simulink model "SimpleBotModel"  (R2024a)
settings: Solver=ode15s  StartTime=0.0  StopTime=2  MaxStep=1e-3  MinStep=1e-5  RelTol=1e-6  AbsTol=1e-3
values from neighbouring files (symbols this model uses):
  Achsabstand = 0.15    [Model1Sensibilities.m]    (also in Model1numericalPSA.m; Model2Sensibilities.m; Modellvalidierung.m; MotorSens2.m)
  B_dis = 0.25    [Model1Sensibilities.m]    (also in Model1numericalPSA.m = 0.15; Model2Sensibilities.m; Modellvalidierung.m = 0.15; MotorSens2.m)
  motor_BackEMFkoef = 0.0035    [Model1Sensibilities.m]    (also in Model1numericalPSA.m; Model2Sensibilities.m; Modellvalidierung.m; MotorSens2.m)
  Motoruebersetzung = 100    [Model1Sensibilities.m]    (also in Model1numericalPSA.m; Model2Sensibilities.m; Modellvalidierung.m; MotorSens2.m)
  Reifen_Radius = 0.04    [Model1Sensibilities.m]    (also in Model1numericalPSA.m; Model2Sensibilities.m; Modellvalidierung.m; MotorSens2.m)
  StartPos = [0.3;0.3]    [Model1Sensibilities.m]    (also in Model1numericalPSA.m; Model2Sensibilities.m; MotorSens2.m; Motor_Sensitivitaet.m)
  Xi = 2/3    (= 0.666666666667)    [Model1Sensibilities.m]    (also in Model1numericalPSA.m = 0.333333333333; Model2Sensibilities.m; Modellvalidierung.m = 0.333333333333; MotorSens2.m)
  Zielpunkt = [1;1.2]    [Model2Sensibilities.m]    (also in MotorSens2.m; Motor_Sensitivitaet.m; Parameter.m; ParamsModell.m)
libraries: slpidlib x2, simulink x1, mobileRoboticsLib x1
settings Model: Creator=jakob  LastModifiedBy=jakob

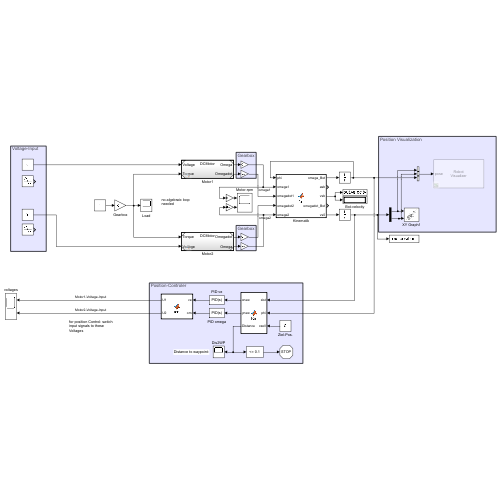
[thumbnail: Simulink's stored preview of the top-level diagram]
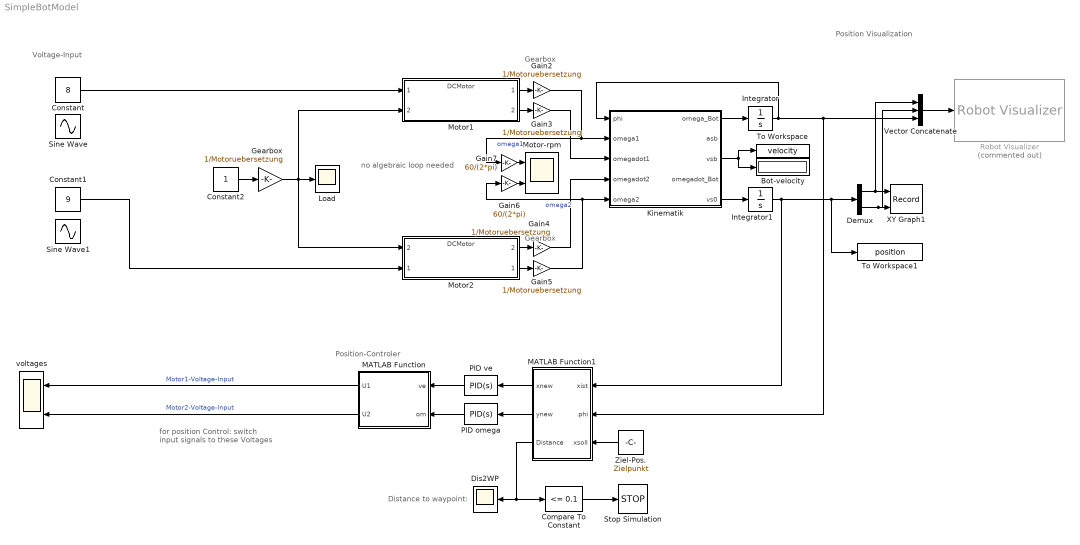
== system SimpleBotModel ==
  note: no algebraic loop needed
  note: Distance to waypoint:
  note: for position Control: switch input signals to these Voltages
  note: Position-Controler
  note: Gearbox
  note: Position Visualization
  note: Voltage-Input
  note: Gearbox
  Bot-velocity : Display
  Compare To Constant : simulink/Logic and Bit Operations/Compare To Constant  relop=<=  const=0.1  OutDataTypeStr=boolean
  Constant : Constant  Value=8  SampleTime=1
  Constant1 : Constant  Value=9  SampleTime=1
  Constant2 : Constant
  Demux : Demux  Outputs=2
  Dis2WP : Scope
  Gain{2..5} (4 alike) : Gain  Gain=1/Motoruebersetzung
  Gain6 : Gain  Gain=60/(2*pi)
  Gain7 : Gain  Gain=60/(2*pi)
  Gearbox : Gain  Gain=1/Motoruebersetzung
  Integrator : Integrator
  Integrator1 : Integrator  InitialCondition=StartPos
  Kinematik : MATLAB Function  TreatAsAtomicUnit=on
  Load : Scope
  MATLAB Function : MATLAB Function  TreatAsAtomicUnit=on
  MATLAB Function1 : MATLAB Function  TreatAsAtomicUnit=on
  Motor-rpm : Scope  NumInputPorts=2
  Motor1 : ModelReference  ModelNameDialog=DCMotor  SimulationMode=Normal  ModelReferenceVersion=1.19
  Motor2 : ModelReference  ModelNameDialog=DCMotor  SimulationMode=Normal  ModelReferenceVersion=1.19
      settings: PortSchema="{\"entries\":[{\"content\":{\"sides\":[{\"content\":{\"connectorIds\":[\"In2\",\"In1\"]},\"type\":\"ConnectorPlacement.EquallySpacedRectSide\",\"uuid\":\"a74839e0-9594-4d91-a47a-bf9c9b4b98c9\"},{\"content\":{\"connectorIds\":[\"Out2\",\"Out1\"],\"side\":\"RIGHT\"},\"type\":\"ConnectorPlacement.EquallySpacedRectSide\",\"uuid\":\"51af5672-9c33-4899-a42f-4b737d1c3e1f\"},{\"content\":{\"side\":\"TOP\"},\"type\":\"ConnectorPlacement.EquallySpacedRectSide\",\"uuid\":\"938b8719-7670-4eda-aa86-bdd9d1e4edbf\"}]},\"type\":\"ConnectorPlacement.EquallySpacedConnector\",\"uuid\":\"899e2604-6c92-4fa5-991d-253a33e61c0b\"}],\"packageUris\":[\"http://schema.mathworks.com/mf0/Connector/R2020b\"],\"version\":\"1.0\"}"
  PID omega : slpidlib/PID Controller  Controller=PID  Form=Parallel  TimeDomain=Continuous-time  UseExternalTs=off  SampleTime=-1  IntegratorMethod=Forward Euler  FilterMethod=Forward Euler  ControllerParametersSource=internal  P=-0.000115423709214701  I=-7.06707739642606e-05  UseKiTs=off  D=-2.53909174243812e-05  UseExternalDerivativeSource=off  N=745.689488508437  UseFilter=on  TunerSelectOption=Transfer Function Based (PID Tuner App)  InitialConditionSource=internal  InitialConditionForIntegrator=0  InitialConditionForFilter=0  DifferentiatorICPrevScaledInput=0  ExternalReset=none  TrackingMode=off  Kt=1  LimitOutput=off  SatLimitsSource=internal  UpperSaturationLimit=inf  LowerSaturationLimit=-inf  LinearizeAsGain=on  AntiWindupMode=none  Kb=1  LimitIntegrator=off  UpperIntegratorSaturationLimit=inf  LowerIntegratorSaturationLimit=-inf  POutMin=[]  POutMax=[]  IOutMin=[]  IOutMax=[]  DOutMin=[]  DOutMax=[]  NOutMin=[]  NOutMax=[]  SumOutMin=[]  SumOutMax=[]  SaturationOutMin=[]  SaturationOutMax=[]  PParamMin=[]  PParamMax=[]  IParamMin=[]  IParamMax=[]  DParamMin=[]  DParamMax=[]  NParamMin=[]  NParamMax=[]  KbParamMin=[]  KbParamMax=[]  KtParamMin=[]  KtParamMax=[]  KbOutMin=[]  KbOutMax=[]  KtOutMin=[]  KtOutMax=[]  IntegratorOutMin=[]  IntegratorOutMax=[]  FilterOutMin=[]  FilterOutMax=[]  SumI1OutMin=[]  SumI1OutMax=[]  SumI2OutMin=[]  SumI2OutMax=[]  SumI3OutMin=[]  SumI3OutMax=[]  SumI4OutMin=[]  SumI4OutMax=[]  SumDOutMin=[]  SumDOutMax=[]  DifferentiatorOutMin=[]  DifferentiatorOutMax=[]  FilterDiffOutCoefMin=[]  FilterDiffOutCoefMax=[]  ReciprocalOutMin=[]  ReciprocalOutMax=[]  SumDenOutMin=[]  SumDenOutMax=[]  SumNumOutMin=[]  SumNumOutMax=[]  DivideOutMin=[]  DivideOutMax=[]  UdiffTsProdOutMin=[]  UdiffTsProdOutMax=[]  NTsProdOutMin=[]  NTsProdOutMax=[]  UintegralTsProdOutMin=[]  UintegralTsProdOutMax=[]  UngainTsProdOutMin=[]  UngainTsProdOutMax=[]  ClampingZeroOutDataTypeStr=Inherit: Inherit via back propagation  ClampingZeroOutMin=[]  ClampingZeroOutMax=[]  FilterDenConstantOutDataTypeStr=Inherit: Inherit via back propagation  FilterDenConstantOutMin=[]  FilterDenConstantOutMax=[]  PCopyOutDataTypeStr=Inherit: Inherit via back propagation  PCopyOutMin=[]  PCopyOutMax=[]  NCopyOutDataTypeStr=Inherit: Inherit via back propagation  NCopyOutMin=[]  NCopyOutMax=[]  IntegratorContinuousStateAttributes=''  IntegratorStateMustResolveToSignalObject=off  IntegratorRTWStateStorageClass=Auto  FilterContinuousStateAttributes=''  FilterStateMustResolveToSignalObject=off  FilterRTWStateStorageClass=Auto  ParallelPVariant=InternalParameters  IdealPVariant=Disabled  IVariant=InternalParameters  DVariant=InternalParameters  IntegratorVariant=Continuous  SatVariant=Disabled  AWVariant=Passthrough  PCopyVariant=Disabled  TRVariant=Disabled  FdbkBlocksVariant=Forward  IdealPFdbkVariant=Disabled  SatFdbkVariant=Disabled  DerivativeFilterVariant=ContFilter  NVariant=InternalParameters  NCopyVariant=Disabled  FilterICVariant=InternalICsFilter  IntegratorICVariant=InternalICs  ExternalResetVariant=Disabled  TRSumVariant=Passthrough  SumFdbkVariant=Disabled  SumVariant=Sum_PID  TsampFilterVariant=InternalTs  TsampNgainVariant=Passthrough  TsampIntegralVariant=Disabled_SignalSpec  ExternalSaturationOutDataTypeStr=Inherit: Same as second input  DerivativeSourceVariant=ErrorSignal
  PID ve : slpidlib/PID Controller  Controller=PID  Form=Parallel  TimeDomain=Continuous-time  UseExternalTs=off  SampleTime=-1  IntegratorMethod=Forward Euler  FilterMethod=Forward Euler  ControllerParametersSource=internal  P=-1.78753184772659e-05  I=-4.36691595478742e-06  UseKiTs=off  D=-2.50467054457144e-06  UseExternalDerivativeSource=off  N=157.882792170406  UseFilter=on  TunerSelectOption=Transfer Function Based (PID Tuner App)  InitialConditionSource=internal  InitialConditionForIntegrator=0  InitialConditionForFilter=0  DifferentiatorICPrevScaledInput=0  ExternalReset=none  TrackingMode=off  Kt=1  LimitOutput=off  SatLimitsSource=internal  UpperSaturationLimit=inf  LowerSaturationLimit=-inf  LinearizeAsGain=on  AntiWindupMode=none  Kb=1  LimitIntegrator=off  UpperIntegratorSaturationLimit=inf  LowerIntegratorSaturationLimit=-inf  POutMin=[]  POutMax=[]  IOutMin=[]  IOutMax=[]  DOutMin=[]  DOutMax=[]  NOutMin=[]  NOutMax=[]  SumOutMin=[]  SumOutMax=[]  SaturationOutMin=[]  SaturationOutMax=[]  PParamMin=[]  PParamMax=[]  IParamMin=[]  IParamMax=[]  DParamMin=[]  DParamMax=[]  NParamMin=[]  NParamMax=[]  KbParamMin=[]  KbParamMax=[]  KtParamMin=[]  KtParamMax=[]  KbOutMin=[]  KbOutMax=[]  KtOutMin=[]  KtOutMax=[]  IntegratorOutMin=[]  IntegratorOutMax=[]  FilterOutMin=[]  FilterOutMax=[]  SumI1OutMin=[]  SumI1OutMax=[]  SumI2OutMin=[]  SumI2OutMax=[]  SumI3OutMin=[]  SumI3OutMax=[]  SumI4OutMin=[]  SumI4OutMax=[]  SumDOutMin=[]  SumDOutMax=[]  DifferentiatorOutMin=[]  DifferentiatorOutMax=[]  FilterDiffOutCoefMin=[]  FilterDiffOutCoefMax=[]  ReciprocalOutMin=[]  ReciprocalOutMax=[]  SumDenOutMin=[]  SumDenOutMax=[]  SumNumOutMin=[]  SumNumOutMax=[]  DivideOutMin=[]  DivideOutMax=[]  UdiffTsProdOutMin=[]  UdiffTsProdOutMax=[]  NTsProdOutMin=[]  NTsProdOutMax=[]  UintegralTsProdOutMin=[]  UintegralTsProdOutMax=[]  UngainTsProdOutMin=[]  UngainTsProdOutMax=[]  ClampingZeroOutDataTypeStr=Inherit: Inherit via back propagation  ClampingZeroOutMin=[]  ClampingZeroOutMax=[]  FilterDenConstantOutDataTypeStr=Inherit: Inherit via back propagation  FilterDenConstantOutMin=[]  FilterDenConstantOutMax=[]  PCopyOutDataTypeStr=Inherit: Inherit via back propagation  PCopyOutMin=[]  PCopyOutMax=[]  NCopyOutDataTypeStr=Inherit: Inherit via back propagation  NCopyOutMin=[]  NCopyOutMax=[]  IntegratorContinuousStateAttributes=''  IntegratorStateMustResolveToSignalObject=off  IntegratorRTWStateStorageClass=Auto  FilterContinuousStateAttributes=''  FilterStateMustResolveToSignalObject=off  FilterRTWStateStorageClass=Auto  ParallelPVariant=InternalParameters  IdealPVariant=Disabled  IVariant=InternalParameters  DVariant=InternalParameters  IntegratorVariant=Continuous  SatVariant=Disabled  AWVariant=Passthrough  PCopyVariant=Disabled  TRVariant=Disabled  FdbkBlocksVariant=Forward  IdealPFdbkVariant=Disabled  SatFdbkVariant=Disabled  DerivativeFilterVariant=ContFilter  NVariant=InternalParameters  NCopyVariant=Disabled  FilterICVariant=InternalICsFilter  IntegratorICVariant=InternalICs  ExternalResetVariant=Disabled  TRSumVariant=Passthrough  SumFdbkVariant=Disabled  SumVariant=Sum_PID  TsampFilterVariant=InternalTs  TsampNgainVariant=Passthrough  TsampIntegralVariant=Disabled_SignalSpec  ExternalSaturationOutDataTypeStr=Inherit: Same as second input  DerivativeSourceVariant=ErrorSignal
  Robot Visualizer : mobileRoboticsLib/Environments/Robot Visualizer  Commented=on  robotRadius=0.1  mapName=myMap  showTrajectory=on  hasWaypoints=off  hasLidar=off  sensorOffset=[ 0, 0 ]  scanAngles=[ -pi/4, 0, pi/4 ]  hasObjDetector=off  objDetectorOffset=[ 0, 0 ]  objDetectorAngle=0  objDetectorFOV=pi/4  objDetectorMaxRange=5  objectColors=[ 1, 0, 0; 0, 1, 0; 0, 0, 1 ]  objectMarkers=s
  Sine Wave : Sin  Amplitude=4  Bias=8  Frequency=2  SampleTime=0
  Sine Wave1 : Sin  Amplitude=2  Bias=9  Frequency=8  SampleTime=0
  Stop Simulation : Stop
  To Workspace : ToWorkspace  VariableName=velocity  SaveFormat=Timeseries  SampleTime=-1
  To Workspace1 : ToWorkspace  VariableName=position  SaveFormat=Timeseries  SampleTime=-1
  Vector Concatenate : Concatenate  NumInputs=3
  XY Graph1 : Record  FileSettingsInternal="{\"entries\":[{\"content\":{\"excelSettings\":{\"content\":{},\"type\":\"Streamout.ExcelSettings\"}},\"type\":\"Streamout.FileSettingStorage\",\"uuid\":\"\"}],\"packageUris\":[\"http:\\/\\/schema.mathworks.com\\/mf0\\/streamout_blocks\\/R2020a\"],\"version\":\"1.0\"}"  Layout=[1 1]  SignalsInternal="{\"entries\":[{\"content\":{\"signals\":[{\"content\":{\"blockPath\":[],\"dimensions\":[1],\"domain\":\"\",\"lineColor\":\"#a2142f\",\"plots\":[ 1 ],\"port\":1,\"signalID\":1,\"signalName\":\"Demux:1\"},\"type\":\"RecordBlkView.Signal\",\"uuid\":\"\"},{\"content\":{\"blockPath\":[],\"dimensions\":[1],\"domain\":\"\",\"lineColor\":\"#139fff\",\"plots\":[ 1 ],\"port\":2,\"signalID\":2,\"signalName\":\"Demux:2\"},\"type\":\"RecordBlkView.Signal\",\"uuid\":\"\"}]},\"type\":\"RecordBlkView.InputSignals\",\"uuid\":\"\"}],\"packageUris\":[\"http:\\/\\/schema.mathworks.com\\/mf0\\/streamout_blocks\\/R2020a\"],\"version\":\"1.0\"}"  VisualizationBindings="{\"xyplotplugin\":{\"info\":[{\"series\":[{\"bindingParametersList\":[{\"parameter\":\"X-Axis\",\"signalID\":1,\"signalName\":\"Demux:1\"},{\"parameter\":\"Y-Axis\",\"signalID\":2,\"signalName\":\"Demux:2\"}],\"seriesID\":0}],\"subplotID\":1}]}}"  CompatibilityTag=XY
  Ziel-Pos. : Constant  Value=Zielpunkt
  voltages : Scope  NumInputPorts=2
  wires:
  Motor1/2 -> Gain3/1
  Demux/2 -> Vector Concatenate/2, XY Graph1/2
  Demux/1 -> Vector Concatenate/1, XY Graph1/1
  Kinematik/5(vs0) -> Integrator1/1
  Kinematik/1(omega_Bot) -> Integrator/1
  Integrator1/1 -> To Workspace1/1, Demux/1, MATLAB Function1/1(xist)
  MATLAB Function/2(U2) -> voltages/2  "Motor2-Voltage-Input"
  Motor1/1 -> Gain2/1
  Gain3/1 -> Kinematik/3(omegadot1)
  Gain2/1 -> Gain7/1, Kinematik/2(omega1)  "omega1"
  Motor2/2 -> Gain4/1
  Motor2/1 -> Gain5/1
  Gain5/1 -> Gain6/1, Kinematik/5(omega2)  "omega2"
  Gain4/1 -> Kinematik/4(omegadot2)
  Gain7/1 -> Motor-rpm/1
  Gain6/1 -> Motor-rpm/2
  PID omega/1 -> MATLAB Function/2(om)
  MATLAB Function1/2(ynew) -> PID omega/1
  Ziel-Pos./1 -> MATLAB Function1/3(xsoll)
  Integrator/1 -> Kinematik/1(phi), MATLAB Function1/2(phi), Vector Concatenate/3
  MATLAB Function1/1(xnew) -> PID ve/1
  PID ve/1 -> MATLAB Function/1(ve)
  Compare To Constant/1 -> Stop Simulation/1
  MATLAB Function/1(U1) -> voltages/1  "Motor1-Voltage-Input"
  MATLAB Function1/3(Distance) -> Compare To Constant/1, Dis2WP/1
  Kinematik/3(vsb) -> To Workspace/1, Bot-velocity/1
  Gearbox/1 -> Motor2/2, Load/1, Motor1/2
  Constant1/1 -> Motor2/1
  Constant/1 -> Motor1/1
  Vector Concatenate/1 -> Robot Visualizer/1
  Constant2/1 -> Gearbox/1

== matlab function SimpleBotModel/MATLAB Function ==
  data: U1 output; U2 output; ve input; om input; motor_BackEMFkoef parameter; Motoruebersetzung parameter; Achsabstand parameter; Reifen_Radius parameter
function [U1, U2] = fcn(ve, om,motor_BackEMFkoef, Motoruebersetzung, Achsabstand, Reifen_Radius)

U1 = (Motoruebersetzung / motor_BackEMFkoef) * ((ve-om*(Achsabstand/2))/Reifen_Radius);
U2 = (Motoruebersetzung / motor_BackEMFkoef) * ((ve+om*(Achsabstand/2))/Reifen_Radius);

% U1 = max(min(U1, 60), -60);
% U2 = max(min(U2, 60), -60);

== matlab function SimpleBotModel/Kinematik ==
  data: phi input; omega_Bot output; omega1 input; omegadot1 input; omegadot2 input; omega2 input; asb output; vsb output; omegadot_Bot output; vs0 output; B_dis parameter; Achsabstand parameter; Reifen_Radius parameter; Xi parameter
function [omega_Bot, asb, vsb, omegadot_Bot, vs0]= fcn(phi, omega1, omegadot1,omegadot2, omega2, B_dis, Achsabstand, Reifen_Radius, Xi)

%RotPhi = [cosd(phi) -sind(phi); sind(phi) cosd(phi)];
Rotb0 = [cos(phi) -sin(phi); sin(phi) cos(phi)];

% b-> Koordinatensystem von Bot
rs1b = [-B_dis*Xi; Achsabstand/2];
rs2b = [-B_dis*Xi ; -Achsabstand/2];
rs10 = Rotb0 *rs1b;
rs20 = Rotb0 *rs2b;

v1b = omega1 * Reifen_Radius;
v2b = omega2 * Reifen_Radius;
v10 = Rotb0 *[1;0]*v1b;
v20 = Rotb0 *[1;0]*v2b;

vsb =(v1b + v2b)/2;
%rs_dot = RotPhi' * vs;
%rs_dot = [vs(1) * cos(phi); vs(1) * sin(phi)];
vs0 = Rotb0 * [1;0] * vsb;

o_numerator = (v20(1) - v10(1)) * (rs10(2) - rs20(2)) + (v20(2) - v10(2)) * (rs20(1) - rs10(1));
o_denominator = (rs10(2) - rs20(2))^2 + (rs20(1) - rs10(1))^2;
omega_Bot = o_numerator / o_denominator;

a1b = omegadot1 * Reifen_Radius;
a2b = omegadot2 * Reifen_Radius;
a10 = Rotb0 * [1;0] * omegadot1 * Reifen_Radius;
a20 = Rotb0 * [1;0] * omegadot2 * Reifen_Radius;
asb = (a1b+a2b)/2;
%as_bot = RotPhi' * as;
%as_bot = [as(1) * cos(phi); as(1) * sin(phi)];

%odot_numerator = (a20(1) - a10(1) - omega_Bot^2 * (r10(1) - r20(1))) * (r10(2) - r20(2)) + (a20(2) - a10(2) - omega_Bot^2 * (r10(2) - r20(2))) * (r20(1) - r10(1));
odot_numerator = (a20(1) - a10(1))*(rs10(2) - rs20(2)) + (a20(2) - a10(2)) * (rs20(1) - rs10(1)) + omega_Bot^2 * ((rs20(1) - rs10(1))*(rs10(2) - rs20(2)) + (rs20(2) - rs10(2))*(rs20(1) - rs10(1)));
odot_denominator = (rs10(2) - rs20(2))^2 + (rs20(1) - rs10(1))^2;
omegadot_Bot = odot_numerator/odot_denominator;

== matlab function SimpleBotModel/MATLAB Function1 ==
  data: xist input; phi input; xnew output; xsoll input; ynew output; Distance output
function [xnew,ynew, Distance] = fcn(xist,phi,xsoll)

Pos_Error = xist-xsoll;   %Distance to waypoint in global coordinates      

RotPhi = [cos(phi) +sin(phi);-sin(phi) cos(phi)];

E_bot = RotPhi * Pos_Error;
xnew = E_bot(1);        %direct distance to waypoint (on body coordinates)
ynew = E_bot(2);        %lateral distance to waypoint (on body coordinates)

Distance = norm(Pos_Error);
